simulink library "Pitch_TASK_Libs"  (Simulink 8.6)
settings: Solver=VariableStepAuto  SolverMode=SingleTasking  StartTime=0.0  StopTime=10.0  RelTol=1e-3
undefined symbols (not defined in the file or in its folder): M_SM_AUTO_RESET_TIME, M_SM_COUNTER_RESET_TIME
libraries: StandardLib x124, WindLib x7, Pitch_TASK_Libs x4, simulink x2
(part 2 of 2)

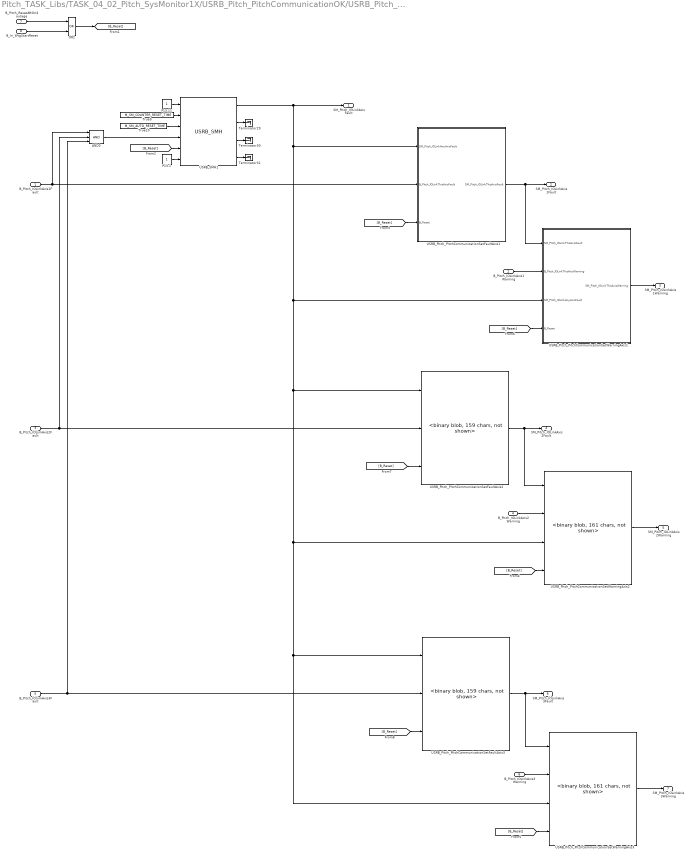
== system Pitch_TASK_Libs/TASK_04_02_Pitch_SysMonitor1X/USRB_Pitch_PitchCommunicationOK/USRB_Pitch_PitchCommunicationSetFaults ==
  B_Pitch_IOLinkAxis1Fault : Inport  OutDataTypeStr=boolean
  B_Pitch_IOLinkAxis1Warning : Inport  Port=2  OutDataTypeStr=boolean
  B_Pitch_IOLinkAxis2Fault : Inport  Port=3  OutDataTypeStr=boolean
  B_Pitch_IOLinkAxis2Warning : Inport  Port=4  OutDataTypeStr=boolean
  B_Pitch_IOLinkAxis3Fault : Inport  Port=5  OutDataTypeStr=boolean
  B_Pitch_IOLinkAxis3Warning : Inport  Port=6  OutDataTypeStr=boolean
  B_Pitch_ResetAftGridoutage : Inport  Port=7  OutDataTypeStr=boolean
  B_In_WtgStartReset : Inport  Port=8  OutDataTypeStr=boolean
  AND3 : StandardLib/Logical operations/AND  RepeatCnt=2  SampleTime=-1  ExecutionOrder=0
  OR2 : StandardLib/Logical operations/OR  RepeatCnt=1  SampleTime=-1  ExecutionOrder=0
  P13.1 : Constant  OutDataTypeStr=boolean  SampleTime=-1
  P13.11 : Constant  OutDataTypeStr=int32  SampleTime=-1
  Terminator29 : Terminator
  Terminator30 : Terminator
  Terminator31 : Terminator
  True10 : Constant  Value=M_SM_AUTO_RESET_TIME  OutDataTypeStr=uint32
  True9 : Constant  Value=M_SM_COUNTER_RESET_TIME  OutDataTypeStr=uint32
  USRB_Pitch_PitchCommunicationSetFaultAxis1 : Subsystem  TreatAsAtomicUnit=on
  USRB_Pitch_PitchCommunicationSetFaultAxis2 : Pitch_TASK_Libs/TASK_04_02_Pitch_SysMonitor2X/USRB_Pitch_PitchCommunicationOK/USRB_Pitch_PitchCommunicationSetFaults/USRB_Pitch_PitchCommunicationSetFaultAxis1  SystemSampleTime=-1
  USRB_Pitch_PitchCommunicationSetFaultAxis3 : Pitch_TASK_Libs/TASK_04_02_Pitch_SysMonitor2X/USRB_Pitch_PitchCommunicationOK/USRB_Pitch_PitchCommunicationSetFaults/USRB_Pitch_PitchCommunicationSetFaultAxis1  SystemSampleTime=-1
  USRB_Pitch_PitchCommunicationSetWarningAxis1 : Subsystem  TreatAsAtomicUnit=on
  USRB_Pitch_PitchCommunicationSetWarningAxis2 : Pitch_TASK_Libs/TASK_04_02_Pitch_SysMonitor2X/USRB_Pitch_PitchCommunicationOK/USRB_Pitch_PitchCommunicationSetFaults/USRB_Pitch_PitchCommunicationSetWarningAxis1  SystemSampleTime=-1
  USRB_Pitch_PitchCommunicationSetWarningAxis3 : Pitch_TASK_Libs/TASK_04_02_Pitch_SysMonitor2X/USRB_Pitch_PitchCommunicationOK/USRB_Pitch_PitchCommunicationSetFaults/USRB_Pitch_PitchCommunicationSetWarningAxis1  SystemSampleTime=-1
  USRB_SMH1 : WindLib/USRB_SMH  Description=|  SystemSampleTime=-1
      | USRB_SMH handles Status Messages. This block sets and resets the Status Message pin SM. There are several possibilitie's to control the reset of SM.                    
      | SM_AUTO_RESET_COUNTS:                                                                                                                                                   
      | Max. number of automatic resets. The resets are counted. If the max. number is reached, the automatic reset is disabled. There exist no limit if the input is set to -1.
      | SM_COUNTER_AUTO_RESET:                                                                                                                                                  
      | This is the time after a automatic reset of the counter is execute.                                                                                                     
      | SM_AUTO_RESET_TIME:                                                                                                                                                     
      | This is the time after a automatic reset of SM is execute.                                                                                                              
      | SM SET:                                                                                                                                                                 
      | Input, that generates a SM. A falling edge is necessary to start the automatic reset function.                                                                          
      | ENABLE:                                                                                                                                                                 
      | Enables the automatic reset function.                                                                                                                                   
      | SM:                                                                                                                                                                     
      | Status Message output.                                                                                                                                                  
      | SM COUNT REACHED:                                                                                                                                                       
      | Shows that the counter reaches the SM AUTO RESET COUNTS                                                                                                                 
      | SM_COUNT:                                                                                                                                                               
      | Actual count of the SM counter
  SM_Pitch_IOLinkAxisFault : Outport  OutDataTypeStr=boolean
  SM_Pitch_IOLinkAxis1Fault : Outport  Port=2  OutDataTypeStr=boolean
  SM_Pitch_IOLinkAxis1Warning : Outport  Port=3  OutDataTypeStr=boolean
  SM_Pitch_IOLinkAxis2Fault : Outport  Port=4  OutDataTypeStr=boolean
  SM_Pitch_IOLinkAxis2Warning : Outport  Port=5  OutDataTypeStr=boolean
  SM_Pitch_IOLinkAxis3Fault : Outport  Port=6  OutDataTypeStr=boolean
  SM_Pitch_IOLinkAxis3Warning : Outport  Port=7  OutDataTypeStr=boolean
  wires:
  [B_Reset] -> USRB_Pitch_PitchCommunicationSetFaultAxis3/3
  B_Pitch_IOLinkAxis3Warning/1 -> USRB_Pitch_PitchCommunicationSetWarningAxis3/2
  [B_Reset] -> USRB_Pitch_PitchCommunicationSetWarningAxis3/4
  USRB_Pitch_PitchCommunicationSetWarningAxis3/1 -> SM_Pitch_IOLinkAxis3Warning/1
  USRB_Pitch_PitchCommunicationSetFaultAxis3/1 -> USRB_Pitch_PitchCommunicationSetWarningAxis3/1, SM_Pitch_IOLinkAxis3Fault/1
  [B_Reset] -> USRB_Pitch_PitchCommunicationSetFaultAxis2/3
  [B_Reset] -> USRB_Pitch_PitchCommunicationSetWarningAxis2/4
  B_Pitch_IOLinkAxis2Warning/1 -> USRB_Pitch_PitchCommunicationSetWarningAxis2/2
  USRB_Pitch_PitchCommunicationSetWarningAxis2/1 -> SM_Pitch_IOLinkAxis2Warning/1
  [B_Reset] -> USRB_Pitch_PitchCommunicationSetWarningAxis1/4(B_Reset)
  B_Pitch_IOLinkAxis1Warning/1 -> USRB_Pitch_PitchCommunicationSetWarningAxis1/2(B_Pitch_IOLinkThisAxisWarning)
  USRB_Pitch_PitchCommunicationSetWarningAxis1/1(SM_Pitch_IOLinkThisAxisWarning) -> SM_Pitch_IOLinkAxis1Warning/1
  USRB_Pitch_PitchCommunicationSetFaultAxis2/1 -> USRB_Pitch_PitchCommunicationSetWarningAxis2/1, SM_Pitch_IOLinkAxis2Fault/1
  USRB_SMH1/1 -> USRB_Pitch_PitchCommunicationSetFaultAxis2/1, USRB_Pitch_PitchCommunicationSetWarningAxis2/3, USRB_Pitch_PitchCommunicationSetWarningAxis3/3, USRB_Pitch_PitchCommunicationSetFaultAxis3/1, USRB_Pitch_PitchCommunicationSetWarningAxis1/3(SM_Pitch_IOLinkAnyAxisFault), USRB_Pitch_PitchCommunicationSetFaultAxis1/1(SM_Pitch_IOLinkAnyAxisFault), SM_Pitch_IOLinkAxisFault/1
  [B_Reset] -> USRB_Pitch_PitchCommunicationSetFaultAxis1/3(B_Reset)
  USRB_Pitch_PitchCommunicationSetFaultAxis1/1(SM_Pitch_IOLinkThisAxisFault) -> USRB_Pitch_PitchCommunicationSetWarningAxis1/1(SM_Pitch_IOLinkThisAxisFault), SM_Pitch_IOLinkAxis1Fault/1
  ? -> ?
  OR2/1 -> [B_Reset]
  [B_Reset] -> USRB_SMH1/5
  B_In_WtgStartReset/1 -> OR2/2
  B_Pitch_ResetAftGridoutage/1 -> OR2/1
  P13.11/1 -> USRB_SMH1/1
  True9/1 -> USRB_SMH1/2
  True10/1 -> USRB_SMH1/3
  P13.1/1 -> USRB_SMH1/6
  USRB_SMH1/2 -> Terminator29/1
  USRB_SMH1/3 -> Terminator30/1
  USRB_SMH1/4 -> Terminator31/1
  AND3/1 -> USRB_SMH1/4
  B_Pitch_IOLinkAxis1Fault/1 -> AND3/1, USRB_Pitch_PitchCommunicationSetFaultAxis1/2(B_Pitch_IOLinkThisAxisFault)
  B_Pitch_IOLinkAxis2Fault/1 -> USRB_Pitch_PitchCommunicationSetFaultAxis2/2, AND3/2
  B_Pitch_IOLinkAxis3Fault/1 -> USRB_Pitch_PitchCommunicationSetFaultAxis3/2, AND3/3

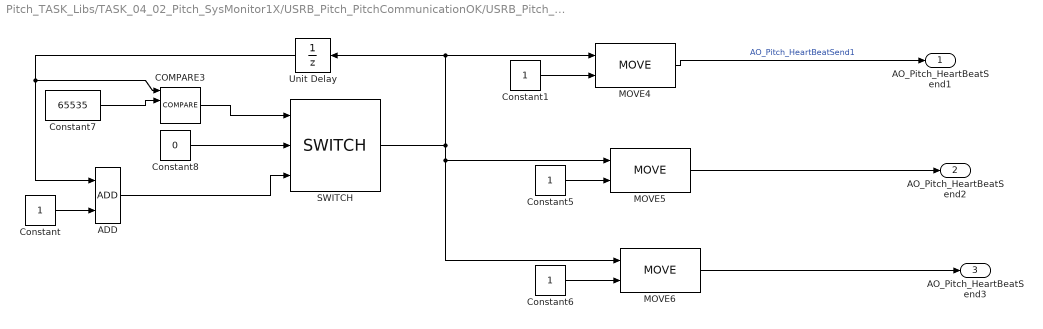
== system Pitch_TASK_Libs/TASK_04_02_Pitch_SysMonitor1X/USRB_Pitch_PitchCommunicationOK/USRB_Pitch_SendHeartbeat ==
  ADD : StandardLib/Math operations/ADD  DataType=INT32  RepeatCnt=1  SampleTime=-1  ExecutionOrder=0
  COMPARE3 : StandardLib/Math operations/COMPARE  Equation=>=  DataType=INT32  SampleTime=-1  ExecutionOrder=0
  Constant : Constant  OutDataTypeStr=int32
  Constant1 : Constant  OutDataTypeStr=boolean
  Constant5 : Constant  OutDataTypeStr=boolean
  Constant6 : Constant  OutDataTypeStr=boolean
  Constant7 : Constant  Value=65535  OutDataTypeStr=int32
  Constant8 : Constant  Value=0  OutDataTypeStr=int32
  MOVE4 : StandardLib/Memory operations/MOVE  DataType=INT32  SampleTime=-1  ExecutionOrder=0
  MOVE5 : StandardLib/Memory operations/MOVE  DataType=INT32  SampleTime=-1  ExecutionOrder=0
  MOVE6 : StandardLib/Memory operations/MOVE  DataType=INT32  SampleTime=-1  ExecutionOrder=0
  SWITCH : StandardLib/Memory operations/SWITCH  DataType=INT32  SampleTime=-1  ExecutionOrder=0
  Unit Delay : UnitDelay  SampleTime=-1
  AO_Pitch_HeartBeatSend1 : Outport  OutDataTypeStr=int32
  AO_Pitch_HeartBeatSend2 : Outport  Port=2  OutDataTypeStr=int32
  AO_Pitch_HeartBeatSend3 : Outport  Port=3  OutDataTypeStr=int32
  wires:
  SWITCH/1 -> Unit Delay/1, MOVE4/1, MOVE6/1, MOVE5/1
  MOVE6/1 -> AO_Pitch_HeartBeatSend3/1
  MOVE5/1 -> AO_Pitch_HeartBeatSend2/1
  Constant8/1 -> SWITCH/2
  ADD/1 -> SWITCH/3
  COMPARE3/1 -> SWITCH/1
  Constant7/1 -> COMPARE3/2
  Unit Delay/1 -> COMPARE3/1, ADD/1
  Constant/1 -> ADD/2
  MOVE4/1 -> AO_Pitch_HeartBeatSend1/1  "AO_Pitch_HeartBeatSend1"
  Constant1/1 -> MOVE4/2
  Constant5/1 -> MOVE5/2
  Constant6/1 -> MOVE6/2

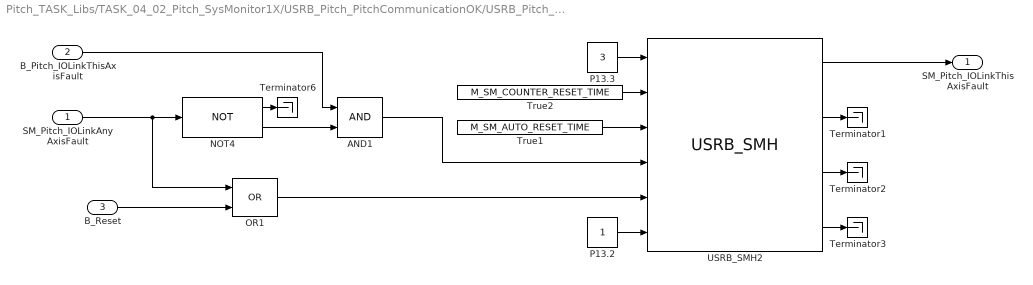
== system Pitch_TASK_Libs/TASK_04_02_Pitch_SysMonitor1X/USRB_Pitch_PitchCommunicationOK/USRB_Pitch_PitchCommunicationSetFaults/USRB_Pitch_PitchCommunicationSetFaultAxis1 ==
  SM_Pitch_IOLinkAnyAxisFault : Inport  OutDataTypeStr=boolean
  B_Pitch_IOLinkThisAxisFault : Inport  Port=2  OutDataTypeStr=boolean
  B_Reset : Inport  Port=3  OutDataTypeStr=boolean
  AND1 : StandardLib/Logical operations/AND  RepeatCnt=1  SampleTime=-1  ExecutionOrder=0
  NOT4 : StandardLib/Logical operations/NOT  SampleTime=-1  ExecutionOrder=0
  OR1 : StandardLib/Logical operations/OR  RepeatCnt=1  SampleTime=-1  ExecutionOrder=0
  P13.2 : Constant  OutDataTypeStr=boolean  SampleTime=-1
  P13.3 : Constant  Value=3  OutDataTypeStr=int32  SampleTime=-1
  Terminator{1..3,6} (4 alike) : Terminator
  True1 : Constant  Value=M_SM_AUTO_RESET_TIME  OutDataTypeStr=uint32
  True2 : Constant  Value=M_SM_COUNTER_RESET_TIME  OutDataTypeStr=uint32
  USRB_SMH2 : WindLib/USRB_SMH  Description=|  SystemSampleTime=-1
      | USRB_SMH handles Status Messages. This block sets and resets the Status Message pin SM. There are several possibilitie's to control the reset of SM.                    
      | SM_AUTO_RESET_COUNTS:                                                                                                                                                   
      | Max. number of automatic resets. The resets are counted. If the max. number is reached, the automatic reset is disabled. There exist no limit if the input is set to -1.
      | SM_COUNTER_AUTO_RESET:                                                                                                                                                  
      | This is the time after a automatic reset of the counter is execute.                                                                                                     
      | SM_AUTO_RESET_TIME:                                                                                                                                                     
      | This is the time after a automatic reset of SM is execute.                                                                                                              
      | SM SET:                                                                                                                                                                 
      | Input, that generates a SM. A falling edge is necessary to start the automatic reset function.                                                                          
      | ENABLE:                                                                                                                                                                 
      | Enables the automatic reset function.                                                                                                                                   
      | SM:                                                                                                                                                                     
      | Status Message output.                                                                                                                                                  
      | SM COUNT REACHED:                                                                                                                                                       
      | Shows that the counter reaches the SM AUTO RESET COUNTS                                                                                                                 
      | SM_COUNT:                                                                                                                                                               
      | Actual count of the SM counter
  SM_Pitch_IOLinkThisAxisFault : Outport  OutDataTypeStr=boolean
  wires:
  B_Reset/1 -> OR1/2
  NOT4/2 -> AND1/2
  NOT4/1 -> Terminator6/1
  B_Pitch_IOLinkThisAxisFault/1 -> AND1/1
  AND1/1 -> USRB_SMH2/4
  OR1/1 -> USRB_SMH2/5
  SM_Pitch_IOLinkAnyAxisFault/1 -> OR1/1, NOT4/1
  P13.3/1 -> USRB_SMH2/1
  True2/1 -> USRB_SMH2/2
  True1/1 -> USRB_SMH2/3
  P13.2/1 -> USRB_SMH2/6
  USRB_SMH2/1 -> SM_Pitch_IOLinkThisAxisFault/1
  USRB_SMH2/2 -> Terminator1/1
  USRB_SMH2/3 -> Terminator2/1
  USRB_SMH2/4 -> Terminator3/1

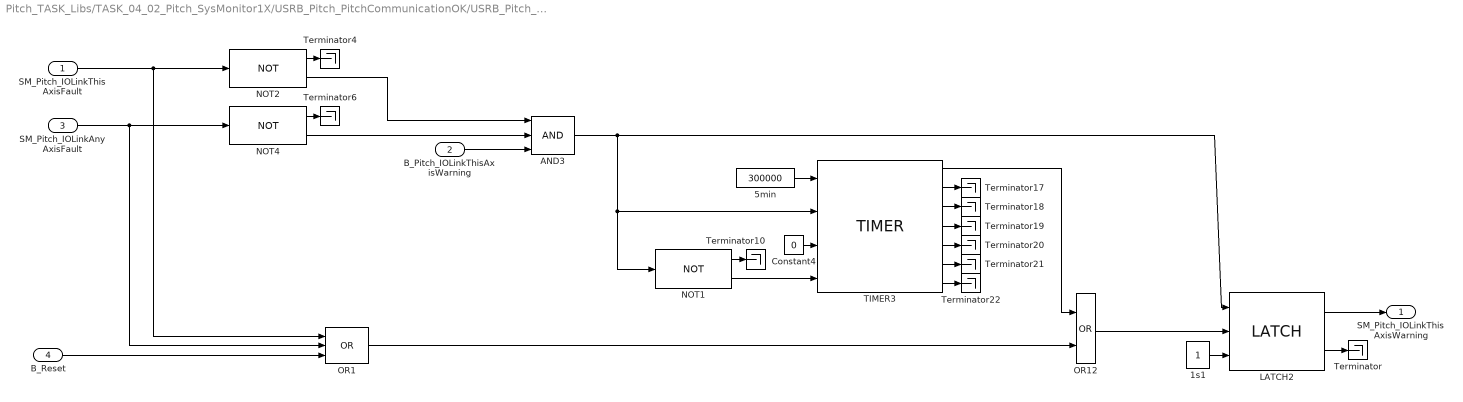
== system Pitch_TASK_Libs/TASK_04_02_Pitch_SysMonitor1X/USRB_Pitch_PitchCommunicationOK/USRB_Pitch_PitchCommunicationSetFaults/USRB_Pitch_PitchCommunicationSetWarningAxis1 ==
  SM_Pitch_IOLinkThisAxisFault : Inport  OutDataTypeStr=boolean
  B_Pitch_IOLinkThisAxisWarning : Inport  Port=2  OutDataTypeStr=boolean
  SM_Pitch_IOLinkAnyAxisFault : Inport  Port=3  OutDataTypeStr=boolean
  B_Reset : Inport  Port=4  OutDataTypeStr=boolean
  1s1 : Constant  VectorParams1D=off  OutDataTypeStr=boolean  SampleTime=-1
  5min : Constant  Value=300000  OutDataTypeStr=uint32  SampleTime=-1
  AND3 : StandardLib/Logical operations/AND  RepeatCnt=2  SampleTime=-1  ExecutionOrder=0
  Constant4 : Constant  Value=0  OutDataTypeStr=boolean
  LATCH2 : StandardLib/Logical operations/LATCH  SampleTime=-1  ExecutionOrder=0
  NOT1 : StandardLib/Logical operations/NOT  SampleTime=-1  ExecutionOrder=0
  NOT2 : StandardLib/Logical operations/NOT  SampleTime=-1  ExecutionOrder=0
  NOT4 : StandardLib/Logical operations/NOT  SampleTime=-1  ExecutionOrder=0
  OR1 : StandardLib/Logical operations/OR  RepeatCnt=2  SampleTime=-1  ExecutionOrder=0
  OR12 : StandardLib/Logical operations/OR  RepeatCnt=1  SampleTime=-1  ExecutionOrder=0
  TIMER3 : StandardLib/Timers and Counters/TIMER  SampleTime=-1  ExecutionOrder=0
  Terminator{,4,6,10,17..22} (10 alike) : Terminator
  SM_Pitch_IOLinkThisAxisWarning : Outport  OutDataTypeStr=boolean
  wires:
  B_Reset/1 -> OR1/3
  SM_Pitch_IOLinkThisAxisFault/1 -> OR1/1, NOT2/1
  SM_Pitch_IOLinkAnyAxisFault/1 -> OR1/2, NOT4/1
  OR12/1 -> LATCH2/2
  TIMER3/1 -> OR12/1
  AND3/1 -> LATCH2/1, NOT1/1, TIMER3/2
  5min/1 -> TIMER3/1
  1s1/1 -> LATCH2/3
  LATCH2/2 -> Terminator/1
  NOT1/1 -> Terminator10/1
  Constant4/1 -> TIMER3/3
  TIMER3/2 -> Terminator17/1
  TIMER3/3 -> Terminator18/1
  TIMER3/4 -> Terminator19/1
  TIMER3/5 -> Terminator20/1
  TIMER3/6 -> Terminator21/1
  TIMER3/7 -> Terminator22/1
  LATCH2/1 -> SM_Pitch_IOLinkThisAxisWarning/1
  NOT1/2 -> TIMER3/4
  OR1/1 -> OR12/2
  NOT2/1 -> Terminator4/1
  B_Pitch_IOLinkThisAxisWarning/1 -> AND3/3
  NOT2/2 -> AND3/1
  NOT4/1 -> Terminator6/1
  NOT4/2 -> AND3/2
